simulink model "heat_exchanger"  (R2017b)
settings: Solver=ode1  StartTime=0.0  StopTime=1000.0  FixedStep=10  RelTol=1e-3
values from neighbouring files (symbols this model uses):
  c_w = 4200    [heat_exchanger_script.m]
  c_wym = 2700    [heat_exchanger_script.m]
  F_zco = 0.035    [heat_exchanger_script.m]
  F_zm = 0.015    [heat_exchanger_script.m]
  k_w = 250000    [heat_exchanger_script.m]
  M_co = 3000    [heat_exchanger_script.m]
  M_m = 3000    [heat_exchanger_script.m]
  rho = 1000    [heat_exchanger_script.m]
  T_pco = 50    [heat_exchanger_script.m]
  T_pm_0 = 15    [heat_exchanger_script.m]
  T_zco_0 = 15    [heat_exchanger_script.m]
  T_zm = 70    [heat_exchanger_script.m]
settings Model: Creator=Michal  LastModifiedBy=Michal

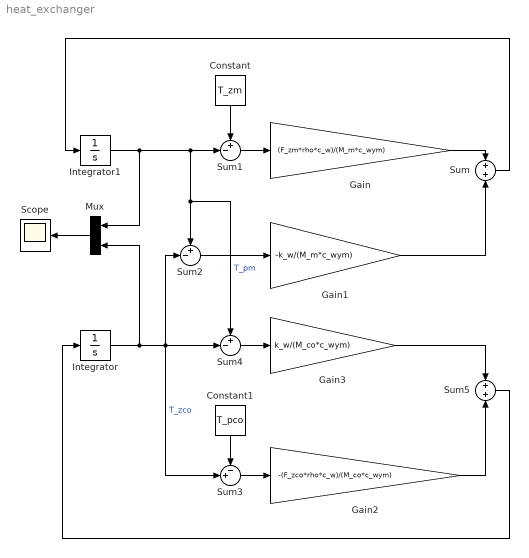
== system heat_exchanger ==
  Constant : Constant  Value=T_zm
  Constant1 : Constant  Value=T_pco
  Gain : Gain  Gain=(F_zm*rho*c_w)/(M_m*c_wym)
  Gain1 : Gain  Gain=-k_w/(M_m*c_wym)
  Gain2 : Gain  Gain=-(F_zco*rho*c_w)/(M_co*c_wym)
  Gain3 : Gain  Gain=k_w/(M_co*c_wym)
  Integrator : Integrator  InitialCondition=T_zco_0
  Integrator1 : Integrator  InitialCondition=T_pm_0
  Mux : Mux  Inputs=2
  Scope : Scope
  Sum : Sum
  Sum1 : Sum  Inputs=+-|
  Sum2 : Sum  Inputs=+-|
  Sum3 : Sum  Inputs=-+|
  Sum4 : Sum  Inputs=+-|
  Sum5 : Sum
  wires:
  Sum1/1 -> Gain/1
  Constant/1 -> Sum1/1
  Gain/1 -> Sum/1
  Integrator1/1 -> Mux/1, Sum4/1, Sum2/1, Sum1/2  "T_pm"
  Integrator/1 -> Mux/2, Sum4/2, Sum3/2, Sum2/2  "T_zco"
  Sum2/1 -> Gain1/1
  Gain1/1 -> Sum/2
  Sum/1 -> Integrator1/1
  Sum3/1 -> Gain2/1
  Constant1/1 -> Sum3/1
  Sum4/1 -> Gain3/1
  Gain3/1 -> Sum5/1
  Gain2/1 -> Sum5/2
  Sum5/1 -> Integrator/1
  Mux/1 -> Scope/1
